simulink model "mRescue"  (R2021a)
settings: Solver=FixedStepAuto  StartTime=0.0  StopTime=inf  RelTol=1e-3  EnableMultiTasking=on
undefined symbols (not defined in the file): adA, adAlpha, adD, adLinkLenghts, adMotorLimits, adOffset
libraries: robotcorelib x1
settings Model: SILPILModeSetting=veronly  ExtModeTrigDuration=2  Creator=angelo  LastModifiedBy=angelo
settings OptimizationCC: EnhancedBackFolding=on  PassReuseOutputArgsAs=Individual arguments  ZeroExternalMemoryAtStartup=off  ZeroInternalMemoryAtStartup=off  MaxStackSize=64  OptimizeBlockOrder=speed  DifferentSizesBufferReuse=on  OptimizationCustomize=off  EfficientTunableParamExpr=on
settings DebuggingCC: ParameterTunabilityLossMsg=error
settings HardwareCC: ProdBitPerInt=16  ProdBitPerPointer=16  ProdBitPerSizeT=16  ProdBitPerPtrDiffT=16  ProdLargestAtomicFloat=None  ProdWordSize=8  ProdHWDeviceType=Atmel->AVR
settings SFSimCC: MATLABDynamicMemAlloc=off
settings RTWCC: SystemTargetFile=ert.tlc  HardwareBoard=Arduino Mega 2560  TemplateMakefile=ert_default_tmf  Toolchain=Arduino AVR  BuildConfiguration=Faster Runs
settings CodeAppCC: ForceParamTrailComments=on  IgnoreCustomStorageClasses=off  OperatorAnnotations=on  SimulinkDataObjDesc=on  SFDataObjDesc=on  InsertBlockDesc=on
settings ERTTargetCC: SupportContinuousTime=on  SupportVariableSizeSignals=on  ExtModeStaticAllocSize=2048

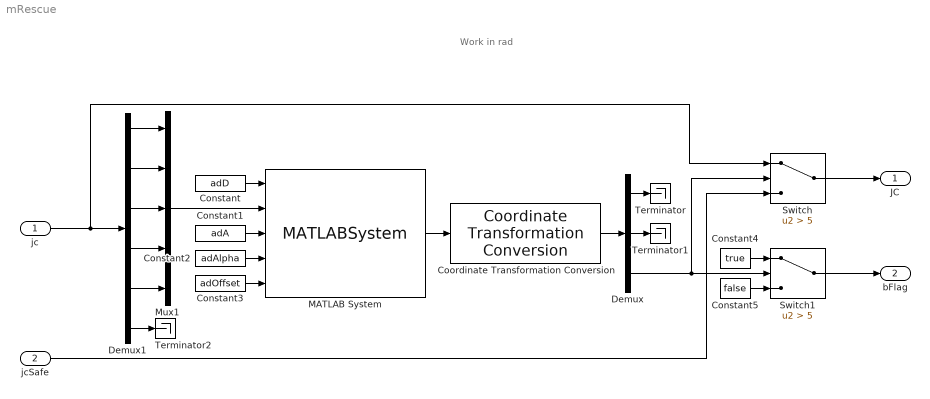
== system mRescue ==
  note: Work in rad
  jc : Inport  PortDimensions=6
  jcSafe : Inport  Port=2  PortDimensions=6
  Constant : Constant  Value=adD
  Constant1 : Constant  Value=adA
  Constant2 : Constant  Value=adAlpha
  Constant3 : Constant  Value=adOffset
  Constant4 : Constant  Value=true
  Constant5 : Constant  Value=false
  Coordinate Transformation Conversion : robotcorelib/Coordinate Transformation Conversion  InputRepresentation=Homogeneous Transformation  InputEulerSequence=ZYX  ShowTrVecInputPort=on  OutputRepresentation=Translation Vector  OutputEulerSequence=ZYX  ShowTrVecOutputPort=on  SimulateUsing=Interpreted execution
      settings: SourceProductBaseCode=NV,RO,RR,UV
  Demux : Demux  Outputs=3
  Demux1 : Demux  Outputs=6
  MATLAB System : MATLABSystem  System=oKINSolver  adHomeDeg=adHome6deg  nGroundLength=adLinkLenghts(1)  nArmLength=adLinkLenghts(2)  nForearmLength=adLinkLenghts(3)  nHandLength=adLinkLenghts(4)  adBaseMinMaxDeg=adMotorLimits(1,:)  adShoulderMinMaxDeg=adMotorLimits(2,:)  adElbowMinMaxDeg=adMotorLimits(3,:)  adPitchMinMaxDeg=adMotorLimits(4,:)  adRollMinMaxDeg=adMotorLimits(5,:)  SimulateUsing=Code generation
      mask Type: oKINSolver
      mask Display:
      | disp('oKINSolver');
      | port_label('input',1,'adD');
      | port_label('input',2,'adQ');
      | port_label('input',3,'adA');
      | port_label('input',4,'adAlpha');
      | port_label('input',5,'adOffset');
      | port_label('output',1,'adPoint');
  Mux1 : Mux  Inputs=5
  Switch : Switch  Criteria=u2 > Threshold  Threshold=5
  Switch1 : Switch  Criteria=u2 > Threshold  Threshold=5
  Terminator : Terminator
  Terminator1 : Terminator
  Terminator2 : Terminator
  JC : Outport
  bFlag : Outport  Port=2
  wires:
  Coordinate Transformation Conversion/1 -> Demux/1
  Demux/1 -> Terminator/1
  Demux/2 -> Terminator1/1
  Switch/1 -> JC/1
  Constant/1 -> MATLAB System/1
  Constant1/1 -> MATLAB System/3
  Constant2/1 -> MATLAB System/4
  Constant3/1 -> MATLAB System/5
  Demux/3 -> Switch/2, Switch1/2
  jcSafe/1 -> Switch/3
  Constant4/1 -> Switch1/1
  Constant5/1 -> Switch1/3
  Switch1/1 -> bFlag/1
  Demux1/1 -> Mux1/1
  Demux1/2 -> Mux1/2
  Demux1/3 -> Mux1/3
  Demux1/4 -> Mux1/4
  Demux1/5 -> Mux1/5
  Demux1/6 -> Terminator2/1
  jc/1 -> Switch/1, Demux1/1
  Mux1/1 -> MATLAB System/2
  MATLAB System/1 -> Coordinate Transformation Conversion/1
